simulink library "environments"  (R2014b)
settings: Solver=ode45  StartTime=0.0  StopTime=10.0  RelTol=1e-3
undefined symbols (not defined in the file): wheel, X, Y, Z
libraries: sm_lib x52, contactlibV2 x20, nesl_utility x4
settings Model: Creator=scastro  LastModifiedBy=scastro

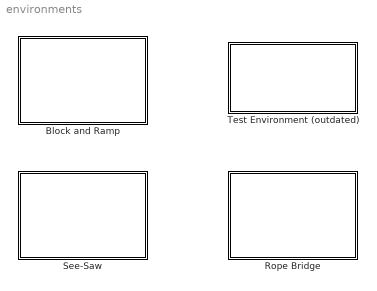
== system environments ==
  Block and Ramp : Subsystem  mask{k=3000, b=25, b2=10}
      mask prompts: k "Contact Stiffness"; b "Contact Damping"; b2 "Friction Damping"
  Rope Bridge : Subsystem  VariantControl=Variant2  mask{k=3000, b=25, b2=10, kbridge=10, dbridge=0.05}
      mask prompts: k "Contact Stiffness"; b "Contact Damping"; b2 "Friction Damping"; kbridge "Bridge Stiffness"; dbridge "Bridge Damping"
  See-Saw : Subsystem  mask{k=3000, b=25, b2=10}
      mask prompts: k "Contact Stiffness"; b "Contact Damping"; b2 "Friction Damping"
  Test Environment (outdated) : Subsystem

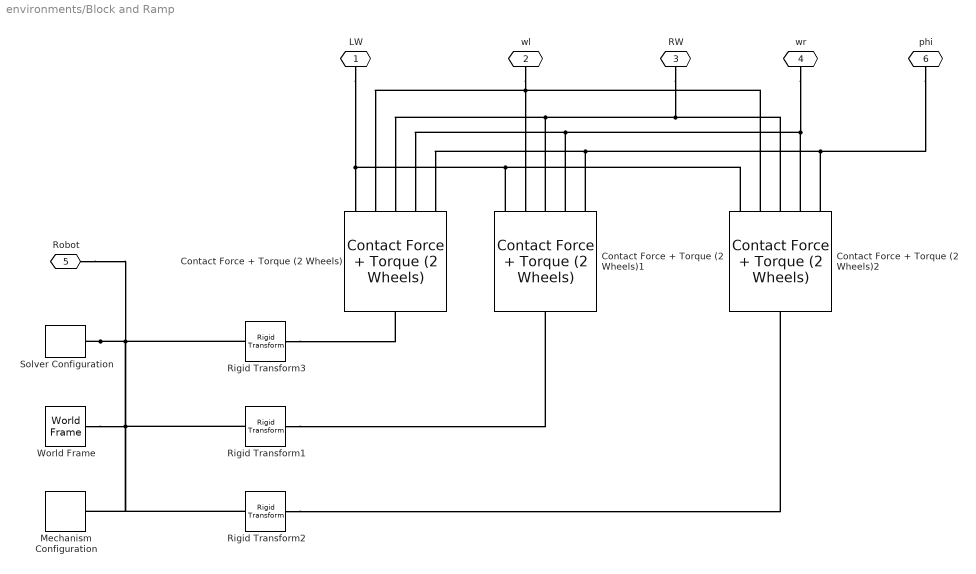
== system environments/Block and Ramp ==
  Contact Force + Torque (2 Wheels) : contactlibV2/Contact Force + Torque (2 Wheels)  rWheel=wheel.r  k=k  b=b  b2=b2  xBlock=3  yBlock=3  zBlock=0.01  mBlock=5  blockColor=[0.2 0.2 1]
  Contact Force + Torque (2 Wheels)1 : contactlibV2/Contact Force + Torque (2 Wheels)  rWheel=wheel.r  k=k  b=b  b2=b2  xBlock=1  yBlock=3  zBlock=0.025  mBlock=5  blockColor=[0.2 0.6 0.2]
  Contact Force + Torque (2 Wheels)2 : contactlibV2/Contact Force + Torque (2 Wheels)  rWheel=wheel.r  k=k  b=b  b2=b2  xBlock=1  yBlock=3  zBlock=0.025  mBlock=5  blockColor=[0.6 0.2 0.2]
  Mechanism Configuration : sm_lib/Utilities/Mechanism Configuration  UniformGravity=Constant  GravityVector=[0 0 -9.80665]  GravityUnits=m/s^2  LinearizationDelta=0.001  BlockFunction=simmechanics.library.utilities.mechanism_configuration
  Rigid Transform1 : sm_lib/Frames and Transforms/Rigid Transform  TranslationMethod=Cartesian  TranslationLengthUnit=m  TranslationStandardAxis=+Z  TranslationStandardOffset=0  TranslationCartesianOffset=[1 0 0.0825-0.12]  TranslationROffset=0  TranslationROffsetUnits=m  TranslationZOffset=0  TranslationZOffsetUnits=m  TranslationThetaOffset=0  TranslationThetaOffsetUnits=deg  RotationMethod=StandardAxis  RotationAngleUnits=deg  RotationStandardAxis=+Z  RotationAngle=0  RotationArbitraryAxis=[0 0 1]  FollAlignAxisA=+X  BaseAlignAxisA=+Y  FollAlignAxisB=+Y  BaseAlignAxisB=+Z  RotationMatrix=[1 0 0; 0 1 0; 0 0 1]  BlockFunction=simmechanics.library.frames_transforms.rigid_transform
  Rigid Transform2 : sm_lib/Frames and Transforms/Rigid Transform  TranslationMethod=Cartesian  TranslationLengthUnit=m  TranslationStandardAxis=+Z  TranslationStandardOffset=0  TranslationCartesianOffset=[-1 0 0.084]  TranslationROffset=0  TranslationROffsetUnits=m  TranslationZOffset=0  TranslationZOffsetUnits=m  TranslationThetaOffset=0  TranslationThetaOffsetUnits=deg  RotationMethod=StandardAxis  RotationAngleUnits=deg  RotationStandardAxis=+Y  RotationAngle=15  RotationArbitraryAxis=[0 0 1]  FollAlignAxisA=+X  BaseAlignAxisA=+Y  FollAlignAxisB=+Y  BaseAlignAxisB=+Z  RotationMatrix=[1 0 0; 0 1 0; 0 0 1]  BlockFunction=simmechanics.library.frames_transforms.rigid_transform
  Rigid Transform3 : sm_lib/Frames and Transforms/Rigid Transform  TranslationMethod=Cartesian  TranslationLengthUnit=m  TranslationStandardAxis=+Z  TranslationStandardOffset=0  TranslationCartesianOffset=[0 0 -(wheel.r+0.01)]  TranslationROffset=0  TranslationROffsetUnits=m  TranslationZOffset=0  TranslationZOffsetUnits=m  TranslationThetaOffset=0  TranslationThetaOffsetUnits=deg  RotationMethod=StandardAxis  RotationAngleUnits=deg  RotationStandardAxis=+Z  RotationAngle=0  RotationArbitraryAxis=[0 0 1]  FollAlignAxisA=+X  BaseAlignAxisA=+Y  FollAlignAxisB=+Y  BaseAlignAxisB=+Z  RotationMatrix=[1 0 0; 0 1 0; 0 0 1]  BlockFunction=simmechanics.library.frames_transforms.rigid_transform
  Solver Configuration : nesl_utility/Solver Configuration  PhysicalDomain=network_engine_domain  SubClassName=solver  LeftPortType=input  RightPortType=generic  Accelerate=off  Tones=[]  Harmonics=[]  SimulateNoise=off  Profile=off  UseLocalSampling=off  EnableSwitchedLinearOptims=on  FrequencyDomain=off  UseCCode=off  RelTol=0.001  AbsTol=1e-06  MinStep=1e-09  ToWorkspace=off  DoDC=off  ResidualTolerance=1e-09  UseLocalSolver=off  LocalSolverChoice=NE_BACKWARD_EULER_ADVANCER  LocalSolverSampleTime=0.001  DoFixedCost=off  MaxNonlinIter=3  MaxModeIter=2  LinearAlgebra=Sparse  DelaysMemoryBudget=1024  AutomaticFiltering=on  FilteringTimeConstant=0.001
  World Frame : sm_lib/Frames and Transforms/World Frame  BlockFunction=simmechanics.library.frames_transforms.world_frame
  LW : PMIOPort  Port=1  Side=Right
  wl : PMIOPort  Port=2  Side=Right
  RW : PMIOPort  Port=3  Side=Right
  wr : PMIOPort  Port=4  Side=Right
  Robot : PMIOPort  Port=5  Side=Left
  phi : PMIOPort  Port=6  Side=Right
  connections:
  Rigid Transform3/RConn1 -- Contact Force + Torque (2 Wheels)/LConn1
  Solver Configuration/RConn1 -- Rigid Transform1/LConn1 -- Mechanism Configuration/RConn1 -- Rigid Transform2/LConn1 -- World Frame/RConn1 -- Robot/RConn1 -- Rigid Transform3/LConn1
  Contact Force + Torque (2 Wheels)1/RConn1 -- Contact Force + Torque (2 Wheels)/RConn1 -- LW/RConn1 -- Contact Force + Torque (2 Wheels)2/RConn1
  Rigid Transform1/RConn1 -- Contact Force + Torque (2 Wheels)1/LConn1
  wl/RConn1 -- Contact Force + Torque (2 Wheels)2/RConn2 -- Contact Force + Torque (2 Wheels)1/RConn2 -- Contact Force + Torque (2 Wheels)/RConn2
  RW/RConn1 -- Contact Force + Torque (2 Wheels)2/RConn3 -- Contact Force + Torque (2 Wheels)1/RConn3 -- Contact Force + Torque (2 Wheels)/RConn3
  wr/RConn1 -- Contact Force + Torque (2 Wheels)2/RConn4 -- Contact Force + Torque (2 Wheels)1/RConn4 -- Contact Force + Torque (2 Wheels)/RConn4
  phi/RConn1 -- Contact Force + Torque (2 Wheels)2/RConn5 -- Contact Force + Torque (2 Wheels)1/RConn5 -- Contact Force + Torque (2 Wheels)/RConn5
  Rigid Transform2/RConn1 -- Contact Force + Torque (2 Wheels)2/LConn1

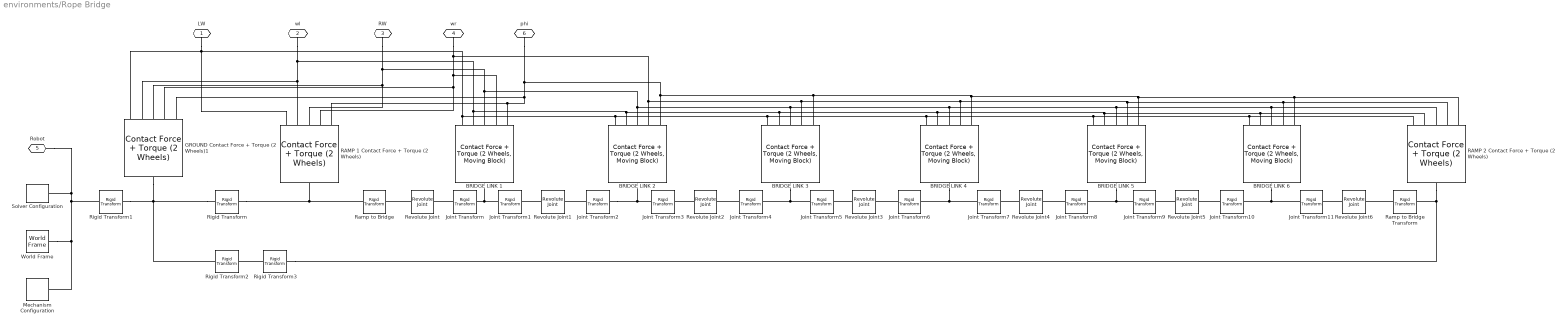
== system environments/Rope Bridge ==
  " BRIDGE LINK 1" : contactlibV2/Contact Force + Torque (2 Wheels, Moving Block)  rWheel=wheel.r  k=k  b=b  b2=b2  xBlock=2.5*(0.0254)  yBlock=12*(0.0254)  zBlock=0.75*(0.0254)  mBlock=0.2  blockColor=[1 0 0]
  " BRIDGE LINK 2" : contactlibV2/Contact Force + Torque (2 Wheels, Moving Block)  rWheel=wheel.r  k=k  b=b  b2=b2  xBlock=2.5*(0.0254)  yBlock=12*(0.0254)  zBlock=0.75*(0.0254)  mBlock=0.2  blockColor=[0 1 0]
  " BRIDGE LINK 3" : contactlibV2/Contact Force + Torque (2 Wheels, Moving Block)  rWheel=wheel.r  k=k  b=b  b2=b2  xBlock=2.5*(0.0254)  yBlock=12*(0.0254)  zBlock=0.75*(0.0254)  mBlock=0.2  blockColor=[1 0 0]
  " BRIDGE LINK 4" : contactlibV2/Contact Force + Torque (2 Wheels, Moving Block)  rWheel=wheel.r  k=k  b=b  b2=b2  xBlock=2.5*(0.0254)  yBlock=12*(0.0254)  zBlock=0.75*(0.0254)  mBlock=0.2  blockColor=[0 1 0]
  " BRIDGE LINK 5" : contactlibV2/Contact Force + Torque (2 Wheels, Moving Block)  rWheel=wheel.r  k=k  b=b  b2=b2  xBlock=2.5*(0.0254)  yBlock=12*(0.0254)  zBlock=0.75*(0.0254)  mBlock=0.2  blockColor=[1 0 0]
  " BRIDGE LINK 6" : contactlibV2/Contact Force + Torque (2 Wheels, Moving Block)  rWheel=wheel.r  k=k  b=b  b2=b2  xBlock=2.5*(0.0254)  yBlock=12*(0.0254)  zBlock=0.75*(0.0254)  mBlock=0.2  blockColor=[0 1 0]
  GROUND Contact Force + Torque (2 Wheels)1 : contactlibV2/Contact Force + Torque (2 Wheels)  rWheel=wheel.r  k=k  b=b  b2=b2  xBlock=24*(0.0254)  yBlock=12*(0.0254)  zBlock=0.5*(0.0254)  mBlock=5  blockColor=[0.2 0.2 0.6]
  Joint Transform : sm_lib/Frames and Transforms/Rigid Transform  TranslationMethod=StandardAxis  TranslationLengthUnit=in  TranslationStandardAxis=+X  TranslationStandardOffset=1.25  TranslationCartesianOffset=[1.25 0 -0.2]  TranslationROffset=0  TranslationROffsetUnits=m  TranslationZOffset=0  TranslationZOffsetUnits=m  TranslationThetaOffset=0  TranslationThetaOffsetUnits=deg  RotationMethod=StandardAxis  RotationAngleUnits=deg  RotationStandardAxis=-X  RotationAngle=90  RotationArbitraryAxis=[0 0 1]  FollAlignAxisA=+X  BaseAlignAxisA=+Y  FollAlignAxisB=+Y  BaseAlignAxisB=+Z  RotationMatrix=[1 0 0; 0 1 0; 0 0 1]  BlockFunction=simmechanics.library.frames_transforms.rigid_transform
  Joint Transform{1,3,5,7,9} (5 alike) : sm_lib/Frames and Transforms/Rigid Transform  TranslationMethod=StandardAxis  TranslationLengthUnit=in  TranslationStandardAxis=+X  TranslationStandardOffset=1.25  TranslationCartesianOffset=[(11*cos(asin(4.75/22))) 0 4.75/2]  TranslationROffset=0  TranslationROffsetUnits=m  TranslationZOffset=0  TranslationZOffsetUnits=m  TranslationThetaOffset=0  TranslationThetaOffsetUnits=deg  RotationMethod=StandardAxis  RotationAngleUnits=deg  RotationStandardAxis=+X  RotationAngle=90  RotationArbitraryAxis=[0 0 1]  FollAlignAxisA=+X  BaseAlignAxisA=+Y  FollAlignAxisB=+Y  BaseAlignAxisB=+Z  RotationMatrix=[1 0 0; 0 1 0; 0 0 1]  BlockFunction=simmechanics.library.frames_transforms.rigid_transform
  Joint Transform{2,4,6,8,10} (5 alike) : sm_lib/Frames and Transforms/Rigid Transform  TranslationMethod=StandardAxis  TranslationLengthUnit=in  TranslationStandardAxis=+X  TranslationStandardOffset=1.25  TranslationCartesianOffset=[(11*cos(asin(4.75/22))) 0 4.75/2]  TranslationROffset=0  TranslationROffsetUnits=m  TranslationZOffset=0  TranslationZOffsetUnits=m  TranslationThetaOffset=0  TranslationThetaOffsetUnits=deg  RotationMethod=StandardAxis  RotationAngleUnits=deg  RotationStandardAxis=-X  RotationAngle=90  RotationArbitraryAxis=[0 0 1]  FollAlignAxisA=+X  BaseAlignAxisA=+Y  FollAlignAxisB=+Y  BaseAlignAxisB=+Z  RotationMatrix=[1 0 0; 0 1 0; 0 0 1]  BlockFunction=simmechanics.library.frames_transforms.rigid_transform
  Joint Transform11 : sm_lib/Frames and Transforms/Rigid Transform  TranslationMethod=Cartesian  TranslationLengthUnit=in  TranslationStandardAxis=+X  TranslationStandardOffset=1.25  TranslationCartesianOffset=[1.25 0 0]  TranslationROffset=0  TranslationROffsetUnits=m  TranslationZOffset=0  TranslationZOffsetUnits=m  TranslationThetaOffset=0  TranslationThetaOffsetUnits=deg  RotationMethod=StandardAxis  RotationAngleUnits=deg  RotationStandardAxis=+X  RotationAngle=90  RotationArbitraryAxis=[0 0 1]  FollAlignAxisA=+X  BaseAlignAxisA=+Y  FollAlignAxisB=+Y  BaseAlignAxisB=+Z  RotationMatrix=[1 0 0; 0 1 0; 0 0 1]  BlockFunction=simmechanics.library.frames_transforms.rigid_transform
  Mechanism Configuration : sm_lib/Utilities/Mechanism Configuration  UniformGravity=Constant  GravityVector=[0 0 -9.80665]  GravityUnits=m/s^2  LinearizationDelta=0.001  BlockFunction=simmechanics.library.utilities.mechanism_configuration
  RAMP 1 Contact Force + Torque (2 Wheels) : contactlibV2/Contact Force + Torque (2 Wheels)  rWheel=wheel.r  k=k  b=b  b2=b2  xBlock=22*(0.0254)  yBlock=12*(0.0254)  zBlock=0.5*(0.0254)  mBlock=5  blockColor=[0.2 0.2 1]
  RAMP 2 Contact Force + Torque (2 Wheels) : contactlibV2/Contact Force + Torque (2 Wheels)  rWheel=wheel.r  k=k  b=b  b2=b2  xBlock=24*(0.0254)  yBlock=12*(0.0254)  zBlock=0.5*(0.0254)  mBlock=5  blockColor=[0.2 0.2 0.6]
  Ramp to Bridge : sm_lib/Frames and Transforms/Rigid Transform  TranslationMethod=Cartesian  TranslationLengthUnit=in  TranslationStandardAxis=+X  TranslationStandardOffset=11  TranslationCartesianOffset=[11 0 -0.1]  TranslationROffset=0  TranslationROffsetUnits=m  TranslationZOffset=0  TranslationZOffsetUnits=m  TranslationThetaOffset=0  TranslationThetaOffsetUnits=deg  RotationMethod=StandardAxis  RotationAngleUnits=deg  RotationStandardAxis=+X  RotationAngle=90  RotationArbitraryAxis=[0 0 1]  FollAlignAxisA=+X  BaseAlignAxisA=+Y  FollAlignAxisB=+Y  BaseAlignAxisB=+Z  RotationMatrix=[1 0 0; 0 1 0; 0 0 1]  BlockFunction=simmechanics.library.frames_transforms.rigid_transform
  Ramp to Bridge Transform : sm_lib/Frames and Transforms/Rigid Transform  TranslationMethod=Cartesian  TranslationLengthUnit=in  TranslationStandardAxis=-X  TranslationStandardOffset=12  TranslationCartesianOffset=[-12 0 -0.1]  TranslationROffset=0  TranslationROffsetUnits=m  TranslationZOffset=0  TranslationZOffsetUnits=m  TranslationThetaOffset=0  TranslationThetaOffsetUnits=deg  RotationMethod=StandardAxis  RotationAngleUnits=deg  RotationStandardAxis=+X  RotationAngle=90  RotationArbitraryAxis=[0 0 1]  FollAlignAxisA=+X  BaseAlignAxisA=+Y  FollAlignAxisB=+Y  BaseAlignAxisB=+Z  RotationMatrix=[1 0 0; 0 1 0; 0 0 1]  BlockFunction=simmechanics.library.frames_transforms.rigid_transform
  Revolute Joint{,1..6} (7 alike) : sm_lib/Joints/Revolute Joint  SenseConstraintForce=off  SenseConstraintForceX=off  SenseConstraintForceY=off  SenseConstraintForceZ=off  SenseConstraintTorque=off  SenseConstraintTorqueX=off  SenseConstraintTorqueY=off  SenseConstraintTorqueZ=off  SenseTotalForce=off  SenseTotalForceX=off  SenseTotalForceY=off  SenseTotalForceZ=off  SenseTotalTorque=off  SenseTotalTorqueX=off  SenseTotalTorqueY=off  SenseTotalTorqueZ=off  CompositeWrenchDir=FollowerOnBase  CompositeWrenchFrame=BaseFrame  EquilibriumPosition=0  EquilibriumPositionUnits=deg  SpringStiffness=kbridge  SpringStiffnessUnits=N*m/rad  DampingCoefficient=dbridge  DampingCoefficientUnits=N*m/(rad/s)  TorqueActuationMode=NoTorque  MotionActuationMode=ComputedMotion  SensePosition=off  SenseVelocity=off  SenseAcceleration=off  SenseTorqueForce=off  PositionTargetValue=0  PositionTargetValueUnits=deg  PositionTargetSpecify=off  PositionTargetPriority=High  VelocityTargetValue=0  VelocityTargetValueUnits=deg/s  VelocityTargetSpecify=off  VelocityTargetPriority=High  BlockFunction=simmechanics.library.joints.revolute_joint
  Rigid Transform : sm_lib/Frames and Transforms/Rigid Transform  TranslationMethod=Cartesian  TranslationLengthUnit=in  TranslationStandardAxis=+Z  TranslationStandardOffset=0  TranslationCartesianOffset=[(12+11*cos(asin(4.75/22))) 0 4.75/2]  TranslationROffset=0  TranslationROffsetUnits=m  TranslationZOffset=0  TranslationZOffsetUnits=m  TranslationThetaOffset=0  TranslationThetaOffsetUnits=deg  RotationMethod=StandardAxis  RotationAngleUnits=rad  RotationStandardAxis=+Y  RotationAngle=-asin(4.75/22)  RotationArbitraryAxis=[0 0 1]  FollAlignAxisA=+X  BaseAlignAxisA=+Y  FollAlignAxisB=+Y  BaseAlignAxisB=+Z  RotationMatrix=[1 0 0; 0 1 0; 0 0 1]  BlockFunction=simmechanics.library.frames_transforms.rigid_transform
  Rigid Transform1 : sm_lib/Frames and Transforms/Rigid Transform  TranslationMethod=Cartesian  TranslationLengthUnit=m  TranslationStandardAxis=+Z  TranslationStandardOffset=0  TranslationCartesianOffset=[0 0.1 -0.05]  TranslationROffset=0  TranslationROffsetUnits=m  TranslationZOffset=0  TranslationZOffsetUnits=m  TranslationThetaOffset=0  TranslationThetaOffsetUnits=deg  RotationMethod=None  RotationAngleUnits=rad  RotationStandardAxis=+Y  RotationAngle=-asin(4.75/22)  RotationArbitraryAxis=[0 0 1]  FollAlignAxisA=+X  BaseAlignAxisA=+Y  FollAlignAxisB=+Y  BaseAlignAxisB=+Z  RotationMatrix=[1 0 0; 0 1 0; 0 0 1]  BlockFunction=simmechanics.library.frames_transforms.rigid_transform
  Rigid Transform2 : sm_lib/Frames and Transforms/Rigid Transform  TranslationMethod=Cartesian  TranslationLengthUnit=in  TranslationStandardAxis=+Z  TranslationStandardOffset=0  TranslationCartesianOffset=[(12+ 22*cos(asin(4.75/22)) + 14.5 + 12*cos(asin(5.875/24)) ) 0 (4.75+ (5.875/2))]  TranslationROffset=0  TranslationROffsetUnits=m  TranslationZOffset=0  TranslationZOffsetUnits=m  TranslationThetaOffset=0  TranslationThetaOffsetUnits=deg  RotationMethod=None  RotationAngleUnits=rad  RotationStandardAxis=+Y  RotationAngle=-asin(4.75/22)  RotationArbitraryAxis=[0 0 1]  FollAlignAxisA=+X  BaseAlignAxisA=+Y  FollAlignAxisB=+Y  BaseAlignAxisB=+Z  RotationMatrix=[1 0 0; 0 1 0; 0 0 1]  BlockFunction=simmechanics.library.frames_transforms.rigid_transform
  Rigid Transform3 : sm_lib/Frames and Transforms/Rigid Transform  TranslationMethod=None  TranslationLengthUnit=in  TranslationStandardAxis=+Z  TranslationStandardOffset=0  TranslationCartesianOffset=[(12+ 11*cos(asin(4.75/22)) + 14.5 + 12*cos(asin(5.875/24)) ) 0 (4.75+5.875)/2]  TranslationROffset=0  TranslationROffsetUnits=m  TranslationZOffset=0  TranslationZOffsetUnits=m  TranslationThetaOffset=0  TranslationThetaOffsetUnits=deg  RotationMethod=StandardAxis  RotationAngleUnits=rad  RotationStandardAxis=+Y  RotationAngle=-asin(5.875/24)  RotationArbitraryAxis=[0 0 1]  FollAlignAxisA=+X  BaseAlignAxisA=+Y  FollAlignAxisB=+Y  BaseAlignAxisB=+Z  RotationMatrix=[1 0 0; 0 1 0; 0 0 1]  BlockFunction=simmechanics.library.frames_transforms.rigid_transform
  Solver Configuration : nesl_utility/Solver Configuration  PhysicalDomain=network_engine_domain  SubClassName=solver  LeftPortType=input  RightPortType=generic  Accelerate=off  Tones=[]  Harmonics=[]  SimulateNoise=off  Profile=off  UseLocalSampling=off  EnableSwitchedLinearOptims=on  FrequencyDomain=off  UseCCode=off  RelTol=0.001  AbsTol=1e-06  MinStep=1e-09  ToWorkspace=off  DoDC=off  ResidualTolerance=1e-09  UseLocalSolver=off  LocalSolverChoice=NE_BACKWARD_EULER_ADVANCER  LocalSolverSampleTime=0.001  DoFixedCost=off  MaxNonlinIter=3  MaxModeIter=2  LinearAlgebra=Sparse  DelaysMemoryBudget=1024  AutomaticFiltering=on  FilteringTimeConstant=0.001
  World Frame : sm_lib/Frames and Transforms/World Frame  BlockFunction=simmechanics.library.frames_transforms.world_frame
  LW : PMIOPort  Port=1  Side=Right
  wl : PMIOPort  Port=2  Side=Right
  RW : PMIOPort  Port=3  Side=Right
  wr : PMIOPort  Port=4  Side=Right
  Robot : PMIOPort  Port=5  Side=Left
  phi : PMIOPort  Port=6  Side=Right
  connections:
  " BRIDGE LINK 5"/RConn5 -- " BRIDGE LINK 4"/RConn5 -- " BRIDGE LINK 3"/RConn5 -- " BRIDGE LINK 2"/RConn5 -- phi/RConn1 -- GROUND Contact Force + Torque (2 Wheels)1/RConn5 -- " BRIDGE LINK 1"/RConn5 -- RAMP 1 Contact Force + Torque (2 Wheels)/RConn5 -- " BRIDGE LINK 6"/RConn5 -- RAMP 2 Contact Force + Torque (2 Wheels)/RConn5
  " BRIDGE LINK 5"/RConn4 -- " BRIDGE LINK 4"/RConn4 -- " BRIDGE LINK 3"/RConn4 -- " BRIDGE LINK 2"/RConn4 -- wr/RConn1 -- " BRIDGE LINK 1"/RConn4 -- GROUND Contact Force + Torque (2 Wheels)1/RConn4 -- RAMP 1 Contact Force + Torque (2 Wheels)/RConn4 -- RAMP 2 Contact Force + Torque (2 Wheels)/RConn4 -- " BRIDGE LINK 6"/RConn4
  " BRIDGE LINK 5"/RConn3 -- " BRIDGE LINK 4"/RConn3 -- " BRIDGE LINK 3"/RConn3 -- " BRIDGE LINK 2"/RConn3 -- " BRIDGE LINK 1"/RConn3 -- RW/RConn1 -- GROUND Contact Force + Torque (2 Wheels)1/RConn3 -- RAMP 1 Contact Force + Torque (2 Wheels)/RConn3 -- RAMP 2 Contact Force + Torque (2 Wheels)/RConn3 -- " BRIDGE LINK 6"/RConn3
  " BRIDGE LINK 5"/RConn2 -- " BRIDGE LINK 4"/RConn2 -- " BRIDGE LINK 3"/RConn2 -- " BRIDGE LINK 2"/RConn2 -- " BRIDGE LINK 1"/RConn2 -- wl/RConn1 -- GROUND Contact Force + Torque (2 Wheels)1/RConn2 -- RAMP 1 Contact Force + Torque (2 Wheels)/RConn2 -- RAMP 2 Contact Force + Torque (2 Wheels)/RConn2 -- " BRIDGE LINK 6"/RConn2
  " BRIDGE LINK 5"/RConn1 -- " BRIDGE LINK 4"/RConn1 -- " BRIDGE LINK 3"/RConn1 -- " BRIDGE LINK 2"/RConn1 -- " BRIDGE LINK 1"/RConn1 -- GROUND Contact Force + Torque (2 Wheels)1/RConn1 -- LW/RConn1 -- RAMP 1 Contact Force + Torque (2 Wheels)/RConn1 -- RAMP 2 Contact Force + Torque (2 Wheels)/RConn1 -- " BRIDGE LINK 6"/RConn1
  Robot/RConn1 -- Solver Configuration/RConn1 -- World Frame/RConn1 -- Mechanism Configuration/RConn1 -- Rigid Transform1/LConn1
  Ramp to Bridge/LConn1 -- Rigid Transform/RConn1 -- RAMP 1 Contact Force + Torque (2 Wheels)/LConn1
  Rigid Transform/LConn1 -- GROUND Contact Force + Torque (2 Wheels)1/LConn1 -- Rigid Transform1/RConn1 -- Rigid Transform2/LConn1
  Joint Transform/RConn1 -- " BRIDGE LINK 1"/LConn1 -- Joint Transform1/LConn1
  Revolute Joint/LConn1 -- Ramp to Bridge/RConn1
  Joint Transform/LConn1 -- Revolute Joint/RConn1
  Revolute Joint1/LConn1 -- Joint Transform1/RConn1
  Joint Transform3/LConn1 -- Joint Transform2/RConn1 -- " BRIDGE LINK 2"/LConn1
  Joint Transform2/LConn1 -- Revolute Joint1/RConn1
  Joint Transform4/LConn1 -- Revolute Joint2/RConn1
  Revolute Joint2/LConn1 -- Joint Transform3/RConn1
  " BRIDGE LINK 3"/LConn1 -- Joint Transform4/RConn1 -- Joint Transform5/LConn1
  " BRIDGE LINK 4"/LConn1 -- Joint Transform6/RConn1 -- Joint Transform7/LConn1
  Revolute Joint3/LConn1 -- Joint Transform5/RConn1
  Joint Transform6/LConn1 -- Revolute Joint3/RConn1
  Joint Transform8/LConn1 -- Revolute Joint4/RConn1
  Revolute Joint4/LConn1 -- Joint Transform7/RConn1
  " BRIDGE LINK 5"/LConn1 -- Joint Transform8/RConn1 -- Joint Transform9/LConn1
  Revolute Joint5/LConn1 -- Joint Transform9/RConn1
  " BRIDGE LINK 6"/LConn1 -- Joint Transform10/RConn1 -- Joint Transform11/LConn1
  Joint Transform10/LConn1 -- Revolute Joint5/RConn1
  Revolute Joint6/LConn1 -- Joint Transform11/RConn1
  Ramp to Bridge Transform/LConn1 -- RAMP 2 Contact Force + Torque (2 Wheels)/LConn1 -- Rigid Transform3/RConn1
  Ramp to Bridge Transform/RConn1 -- Revolute Joint6/RConn1
  Rigid Transform3/LConn1 -- Rigid Transform2/RConn1

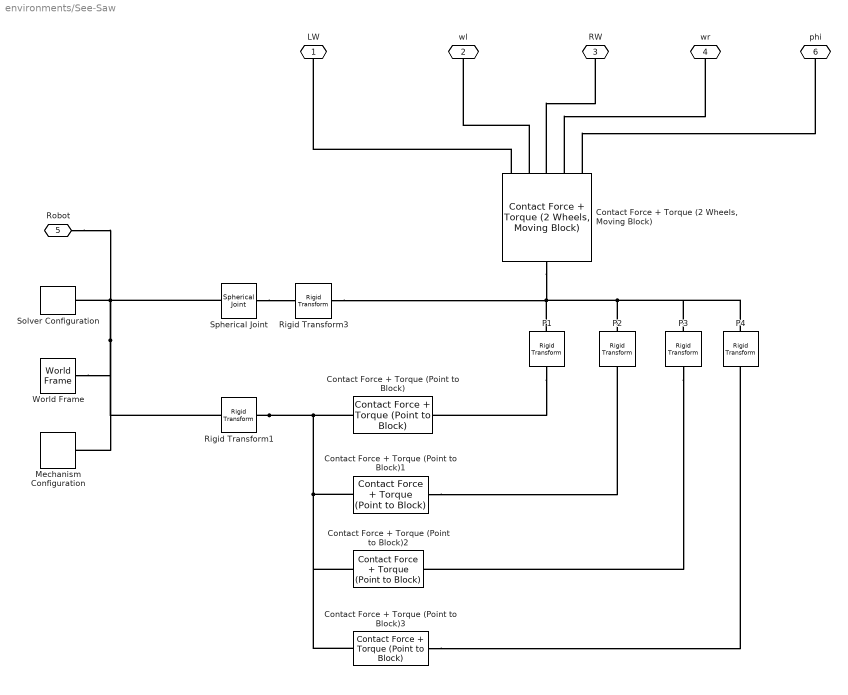
== system environments/See-Saw ==
  "Contact Force + Torque (2 Wheels, Moving Block)" : contactlibV2/Contact Force + Torque (2 Wheels, Moving Block)  rWheel=wheel.r  k=k  b=b  b2=b2  xBlock=2  yBlock=2  zBlock=0.01  mBlock=5  blockColor=[0.2 0.2 1]
  Contact Force + Torque (Point to Block){,1..3} (4 alike) : contactlibV2/Contact Force + Torque (Point to Block)  k=k  b=b  xBlock=5  yBlock=5  zBlock=0.01  mBlock=5  blockColor=[0.2 1 0.2]
  Mechanism Configuration : sm_lib/Utilities/Mechanism Configuration  UniformGravity=Constant  GravityVector=[0 0 -9.80665]  GravityUnits=m/s^2  LinearizationDelta=0.001  BlockFunction=simmechanics.library.utilities.mechanism_configuration
  P1 : sm_lib/Frames and Transforms/Rigid Transform  TranslationMethod=Cartesian  TranslationLengthUnit=m  TranslationStandardAxis=+Z  TranslationStandardOffset=0  TranslationCartesianOffset=[-1 -1 -0.005]  TranslationROffset=0  TranslationROffsetUnits=m  TranslationZOffset=0  TranslationZOffsetUnits=m  TranslationThetaOffset=0  TranslationThetaOffsetUnits=deg  RotationMethod=None  RotationAngleUnits=deg  RotationStandardAxis=-X  RotationAngle=90  RotationArbitraryAxis=[0 0 1]  FollAlignAxisA=+X  BaseAlignAxisA=+Y  FollAlignAxisB=+Y  BaseAlignAxisB=+Z  BlockFunction=simmechanics.library.frames_transforms.rigid_transform
  P2 : sm_lib/Frames and Transforms/Rigid Transform  TranslationMethod=Cartesian  TranslationLengthUnit=m  TranslationStandardAxis=+Z  TranslationStandardOffset=0  TranslationCartesianOffset=[-1 1 -0.005]  TranslationROffset=0  TranslationROffsetUnits=m  TranslationZOffset=0  TranslationZOffsetUnits=m  TranslationThetaOffset=0  TranslationThetaOffsetUnits=deg  RotationMethod=None  RotationAngleUnits=deg  RotationStandardAxis=-X  RotationAngle=90  RotationArbitraryAxis=[0 0 1]  FollAlignAxisA=+X  BaseAlignAxisA=+Y  FollAlignAxisB=+Y  BaseAlignAxisB=+Z  BlockFunction=simmechanics.library.frames_transforms.rigid_transform
  P3 : sm_lib/Frames and Transforms/Rigid Transform  TranslationMethod=Cartesian  TranslationLengthUnit=m  TranslationStandardAxis=+Z  TranslationStandardOffset=0  TranslationCartesianOffset=[1 -1 -0.005]  TranslationROffset=0  TranslationROffsetUnits=m  TranslationZOffset=0  TranslationZOffsetUnits=m  TranslationThetaOffset=0  TranslationThetaOffsetUnits=deg  RotationMethod=None  RotationAngleUnits=deg  RotationStandardAxis=-X  RotationAngle=90  RotationArbitraryAxis=[0 0 1]  FollAlignAxisA=+X  BaseAlignAxisA=+Y  FollAlignAxisB=+Y  BaseAlignAxisB=+Z  BlockFunction=simmechanics.library.frames_transforms.rigid_transform
  P4 : sm_lib/Frames and Transforms/Rigid Transform  TranslationMethod=Cartesian  TranslationLengthUnit=m  TranslationStandardAxis=+Z  TranslationStandardOffset=0  TranslationCartesianOffset=[1 1 -0.005]  TranslationROffset=0  TranslationROffsetUnits=m  TranslationZOffset=0  TranslationZOffsetUnits=m  TranslationThetaOffset=0  TranslationThetaOffsetUnits=deg  RotationMethod=None  RotationAngleUnits=deg  RotationStandardAxis=-X  RotationAngle=90  RotationArbitraryAxis=[0 0 1]  FollAlignAxisA=+X  BaseAlignAxisA=+Y  FollAlignAxisB=+Y  BaseAlignAxisB=+Z  BlockFunction=simmechanics.library.frames_transforms.rigid_transform
  Rigid Transform1 : sm_lib/Frames and Transforms/Rigid Transform  TranslationMethod=Cartesian  TranslationLengthUnit=m  TranslationStandardAxis=+Z  TranslationStandardOffset=0  TranslationCartesianOffset=[0 0 -0.2]  TranslationROffset=0  TranslationROffsetUnits=m  TranslationZOffset=0  TranslationZOffsetUnits=m  TranslationThetaOffset=0  TranslationThetaOffsetUnits=deg  RotationMethod=None  RotationAngleUnits=deg  RotationStandardAxis=-X  RotationAngle=90  RotationArbitraryAxis=[0 0 1]  FollAlignAxisA=+X  BaseAlignAxisA=+Y  FollAlignAxisB=+Y  BaseAlignAxisB=+Z  RotationMatrix=[1 0 0; 0 1 0; 0 0 1]  BlockFunction=simmechanics.library.frames_transforms.rigid_transform
  Rigid Transform3 : sm_lib/Frames and Transforms/Rigid Transform  TranslationMethod=Cartesian  TranslationLengthUnit=m  TranslationStandardAxis=+Z  TranslationStandardOffset=0  TranslationCartesianOffset=[0 0 -(wheel.r+0.01)]  TranslationROffset=0  TranslationROffsetUnits=m  TranslationZOffset=0  TranslationZOffsetUnits=m  TranslationThetaOffset=0  TranslationThetaOffsetUnits=deg  RotationMethod=None  RotationAngleUnits=deg  RotationStandardAxis=-X  RotationAngle=90  RotationArbitraryAxis=[0 0 1]  FollAlignAxisA=+X  BaseAlignAxisA=+Y  FollAlignAxisB=+Y  BaseAlignAxisB=+Z  BlockFunction=simmechanics.library.frames_transforms.rigid_transform
  Solver Configuration : nesl_utility/Solver Configuration  PhysicalDomain=network_engine_domain  SubClassName=solver  LeftPortType=input  RightPortType=generic  Accelerate=off  Tones=[]  Harmonics=[]  SimulateNoise=off  Profile=off  UseLocalSampling=off  EnableSwitchedLinearOptims=on  FrequencyDomain=off  UseCCode=off  RelTol=0.001  AbsTol=1e-06  MinStep=1e-09  ToWorkspace=off  DoDC=off  ResidualTolerance=1e-09  UseLocalSolver=off  LocalSolverChoice=NE_BACKWARD_EULER_ADVANCER  LocalSolverSampleTime=0.001  DoFixedCost=off  MaxNonlinIter=3  MaxModeIter=2  LinearAlgebra=Sparse  DelaysMemoryBudget=1024  AutomaticFiltering=on  FilteringTimeConstant=0.001
  Spherical Joint : sm_lib/Joints/Spherical Joint  SenseConstraintForce=off  SenseConstraintForceX=off  SenseConstraintForceY=off  SenseConstraintForceZ=off  SenseConstraintTorque=off  SenseConstraintTorqueX=off  SenseConstraintTorqueY=off  SenseConstraintTorqueZ=off  SenseTotalForce=off  SenseTotalForceX=off  SenseTotalForceY=off  SenseTotalForceZ=off  SenseTotalTorque=off  SenseTotalTorqueX=off  SenseTotalTorqueY=off  SenseTotalTorqueZ=off  CompositeWrenchDir=FollowerOnBase  CompositeWrenchFrame=BaseFrame  DefPosRotationMethod=None  DefPosRotationAngleUnits=deg  DefPosRotationStandardAxis=+Z  DefPosRotationAngle=0  DefPosRotationArbitraryAxis=[0 0 1]  DefPosFollAlignAxisA=+X  DefPosBaseAlignAxisA=+Y  DefPosFollAlignAxisB=+Y  DefPosBaseAlignAxisB=+Z  DefPosRotationMatrix=[1 0 0; 0 1 0; 0 0 1]  EqPosRotationMethod=None  EqPosRotationAngleUnits=deg  EqPosRotationStandardAxis=+Z  EqPosRotationAngle=0  EqPosRotationArbitraryAxis=[0 0 1]  EqPosFollAlignAxisA=+X  EqPosBaseAlignAxisA=+Y  EqPosFollAlignAxisB=+Y  EqPosBaseAlignAxisB=+Z  EqPosRotationMatrix=[1 0 0; 0 1 0; 0 0 1]  SpringStiffness=12  SpringStiffnessUnits=N*m/rad  DampingCoefficient=1.5  DampingCoefficientUnits=N*m/(rad/s)  ActuateTorqueX=off  ActuateTorqueY=off  ActuateTorqueZ=off  ActuateTorque=off  TorqueActuationMode=NoTorque  MotionActuationMode=ComputedMotion  ActuationFrame=BaseFrame  SensePosition=off  SenseVelocityX=off  SenseVelocityY=off  SenseVelocityZ=off  SenseVelocity=off  SenseAccelerationX=off  SenseAccelerationY=off  SenseAccelerationZ=off  SenseAcceleration=off  SenseTorqueX=off  SenseTorqueY=off  SenseTorqueZ=off  SenseTorqueForce=off  SensingFrame=BaseFrame  PositionTargetRotationMethod=None  PositionTargetRotationAngleUnits=deg  PositionTargetRotationStandardAxis=+Z  PositionTargetRotationAngle=0  PositionTargetRotationArbitraryAxis=[0 0 1]  PositionTargetFollAlignAxisA=+X  PositionTargetBaseAlignAxisA=+Y  PositionTargetFollAlignAxisB=+Y  PositionTargetBaseAlignAxisB=+Z  PositionTargetRotationMatrix=[1 0 0; 0 1 0; 0 0 1]  PositionTargetSpecify=off  PositionTargetPriority=High  VelocityTargetValue=[0 0 0]  VelocityTargetValueUnits=deg/s  VelocityTargetSpecify=off  VelocityTargetPriority=High  VelocityTargetInFollowerFrame=on  BlockFunction=simmechanics.library.joints.spherical_joint
  World Frame : sm_lib/Frames and Transforms/World Frame  BlockFunction=simmechanics.library.frames_transforms.world_frame
  LW : PMIOPort  Port=1  Side=Right
  wl : PMIOPort  Port=2  Side=Right
  RW : PMIOPort  Port=3  Side=Right
  wr : PMIOPort  Port=4  Side=Right
  Robot : PMIOPort  Port=5  Side=Left
  phi : PMIOPort  Port=6  Side=Right
  connections:
  "Contact Force + Torque (2 Wheels, Moving Block)"/RConn5 -- phi/RConn1
  "Contact Force + Torque (2 Wheels, Moving Block)"/RConn4 -- wr/RConn1
  "Contact Force + Torque (2 Wheels, Moving Block)"/RConn3 -- RW/RConn1
  "Contact Force + Torque (2 Wheels, Moving Block)"/RConn2 -- wl/RConn1
  "Contact Force + Torque (2 Wheels, Moving Block)"/RConn1 -- LW/RConn1
  Rigid Transform3/RConn1 -- P4/LConn1 -- P3/LConn1 -- P2/LConn1 -- P1/LConn1 -- "Contact Force + Torque (2 Wheels, Moving Block)"/LConn1
  Robot/RConn1 -- Spherical Joint/LConn1 -- World Frame/RConn1 -- Rigid Transform1/LConn1 -- Mechanism Configuration/RConn1 -- Solver Configuration/RConn1
  Spherical Joint/RConn1 -- Rigid Transform3/LConn1
  Rigid Transform1/RConn1 -- Contact Force + Torque (Point to Block)2/LConn1 -- Contact Force + Torque (Point to Block)3/LConn1 -- Contact Force + Torque (Point to Block)1/LConn1 -- Contact Force + Torque (Point to Block)/LConn1
  P1/RConn1 -- Contact Force + Torque (Point to Block)/RConn1
  Contact Force + Torque (Point to Block)1/RConn1 -- P2/RConn1
  P3/RConn1 -- Contact Force + Torque (Point to Block)2/RConn1
  Contact Force + Torque (Point to Block)3/RConn1 -- P4/RConn1

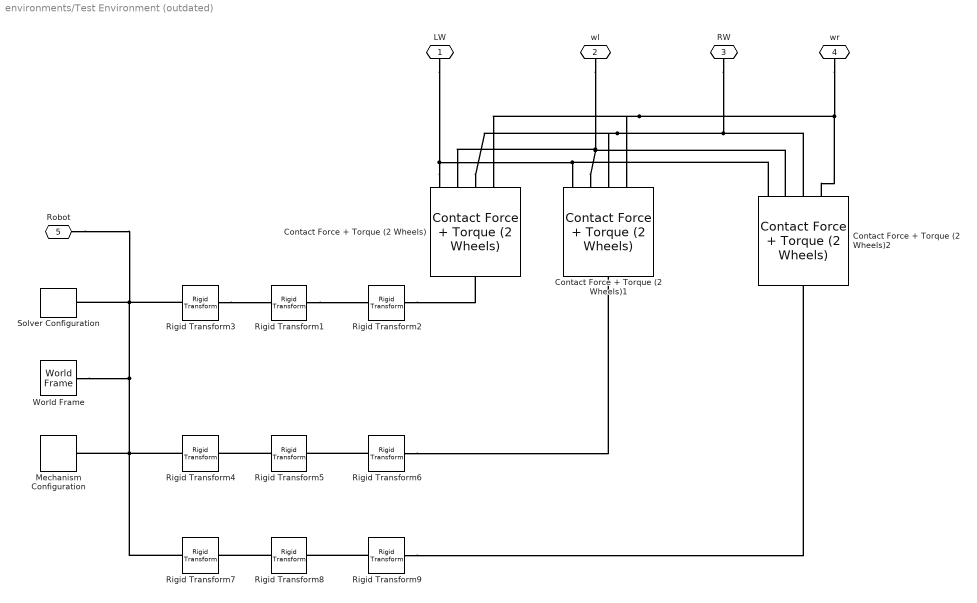
== system environments/Test Environment (outdated) ==
  Contact Force + Torque (2 Wheels) : contactlibV2/Contact Force + Torque (2 Wheels)  rWheel=wheel.r  k=1500  b=25  b2=10  xBlock=3  yBlock=3  zBlock=0.01  mBlock=5  blockColor=[0.2 0.2 1]
  Contact Force + Torque (2 Wheels)1 : contactlibV2/Contact Force + Torque (2 Wheels)  rWheel=wheel.r  k=1500  b=25  b2=10  xBlock=3  yBlock=3  zBlock=0.01  mBlock=5  blockColor=[1 0.2 0.2]
  Contact Force + Torque (2 Wheels)2 : contactlibV2/Contact Force + Torque (2 Wheels)  rWheel=wheel.r  k=1500  b=25  b2=10  xBlock=3  yBlock=3  zBlock=0.01  mBlock=5  blockColor=[0.2 1 0.2]
  Mechanism Configuration : sm_lib/Utilities/Mechanism Configuration  UniformGravity=Constant  GravityVector=[0 0 -9.80665]  GravityUnits=m/s^2  LinearizationDelta=0.001  BlockFunction=simmechanics.library.utilities.mechanism_configuration
  Rigid Transform1 : sm_lib/Frames and Transforms/Rigid Transform  TranslationMethod=None  TranslationLengthUnit=m  TranslationStandardAxis=+Z  TranslationStandardOffset=0  TranslationCartesianOffset=[0 0 -1.25]  TranslationROffset=0  TranslationROffsetUnits=m  TranslationZOffset=0  TranslationZOffsetUnits=m  TranslationThetaOffset=0  TranslationThetaOffsetUnits=deg  RotationMethod=StandardAxis  RotationAngleUnits=deg  RotationStandardAxis=+Y  RotationAngle=5  RotationArbitraryAxis=[0 0 1]  FollAlignAxisA=+X  BaseAlignAxisA=+Y  FollAlignAxisB=+Y  BaseAlignAxisB=+Z  BlockFunction=simmechanics.library.frames_transforms.rigid_transform
  Rigid Transform2 : sm_lib/Frames and Transforms/Rigid Transform  TranslationMethod=None  TranslationLengthUnit=m  TranslationStandardAxis=+Z  TranslationStandardOffset=0  TranslationCartesianOffset=[0 0 -1.25]  TranslationROffset=0  TranslationROffsetUnits=m  TranslationZOffset=0  TranslationZOffsetUnits=m  TranslationThetaOffset=0  TranslationThetaOffsetUnits=deg  RotationMethod=StandardAxis  RotationAngleUnits=deg  RotationStandardAxis=+X  RotationAngle=0  RotationArbitraryAxis=[0 0 1]  FollAlignAxisA=+X  BaseAlignAxisA=+Y  FollAlignAxisB=+Y  BaseAlignAxisB=+Z  BlockFunction=simmechanics.library.frames_transforms.rigid_transform
  Rigid Transform3 : sm_lib/Frames and Transforms/Rigid Transform  TranslationMethod=Cartesian  TranslationLengthUnit=m  TranslationStandardAxis=+Z  TranslationStandardOffset=0  TranslationCartesianOffset=[0 0 -(wheel.r+0.01)]  TranslationROffset=0  TranslationROffsetUnits=m  TranslationZOffset=0  TranslationZOffsetUnits=m  TranslationThetaOffset=0  TranslationThetaOffsetUnits=deg  RotationMethod=StandardAxis  RotationAngleUnits=deg  RotationStandardAxis=+Z  RotationAngle=0  RotationArbitraryAxis=[0 0 1]  FollAlignAxisA=+X  BaseAlignAxisA=+Y  FollAlignAxisB=+Y  BaseAlignAxisB=+Z  RotationMatrix=[1 0 0; 0 1 0; 0 0 1]  BlockFunction=simmechanics.library.frames_transforms.rigid_transform
  Rigid Transform4 : sm_lib/Frames and Transforms/Rigid Transform  TranslationMethod=Cartesian  TranslationLengthUnit=m  TranslationStandardAxis=+Z  TranslationStandardOffset=0  TranslationCartesianOffset=[3 -0 -0.35]  TranslationROffset=0  TranslationROffsetUnits=m  TranslationZOffset=0  TranslationZOffsetUnits=m  TranslationThetaOffset=0  TranslationThetaOffsetUnits=deg  RotationMethod=StandardAxis  RotationAngleUnits=deg  RotationStandardAxis=+Z  RotationAngle=115  RotationArbitraryAxis=[0 0 1]  FollAlignAxisA=+X  BaseAlignAxisA=+Y  FollAlignAxisB=+Y  BaseAlignAxisB=+Z  RotationMatrix=[1 0 0; 0 1 0; 0 0 1]  BlockFunction=simmechanics.library.frames_transforms.rigid_transform
  Rigid Transform5 : sm_lib/Frames and Transforms/Rigid Transform  TranslationMethod=None  TranslationLengthUnit=m  TranslationStandardAxis=+Z  TranslationStandardOffset=0  TranslationCartesianOffset=[0 0 -1.25]  TranslationROffset=0  TranslationROffsetUnits=m  TranslationZOffset=0  TranslationZOffsetUnits=m  TranslationThetaOffset=0  TranslationThetaOffsetUnits=deg  RotationMethod=StandardAxis  RotationAngleUnits=deg  RotationStandardAxis=+Y  RotationAngle=-1  RotationArbitraryAxis=[0 0 1]  FollAlignAxisA=+X  BaseAlignAxisA=+Y  FollAlignAxisB=+Y  BaseAlignAxisB=+Z  BlockFunction=simmechanics.library.frames_transforms.rigid_transform
  Rigid Transform6 : sm_lib/Frames and Transforms/Rigid Transform  TranslationMethod=None  TranslationLengthUnit=m  TranslationStandardAxis=+Z  TranslationStandardOffset=0  TranslationCartesianOffset=[0 0 -1.25]  TranslationROffset=0  TranslationROffsetUnits=m  TranslationZOffset=0  TranslationZOffsetUnits=m  TranslationThetaOffset=0  TranslationThetaOffsetUnits=deg  RotationMethod=StandardAxis  RotationAngleUnits=deg  RotationStandardAxis=+X  RotationAngle=1  RotationArbitraryAxis=[0 0 1]  FollAlignAxisA=+X  BaseAlignAxisA=+Y  FollAlignAxisB=+Y  BaseAlignAxisB=+Z  BlockFunction=simmechanics.library.frames_transforms.rigid_transform
  Rigid Transform7 : sm_lib/Frames and Transforms/Rigid Transform  TranslationMethod=Cartesian  TranslationLengthUnit=m  TranslationStandardAxis=+Z  TranslationStandardOffset=0  TranslationCartesianOffset=[5 -2 -0.55]  TranslationROffset=0  TranslationROffsetUnits=m  TranslationZOffset=0  TranslationZOffsetUnits=m  TranslationThetaOffset=0  TranslationThetaOffsetUnits=deg  RotationMethod=StandardAxis  RotationAngleUnits=deg  RotationStandardAxis=+Z  RotationAngle=0  RotationArbitraryAxis=[0 0 1]  FollAlignAxisA=+X  BaseAlignAxisA=+Y  FollAlignAxisB=+Y  BaseAlignAxisB=+Z  RotationMatrix=[1 0 0; 0 1 0; 0 0 1]  BlockFunction=simmechanics.library.frames_transforms.rigid_transform
  Rigid Transform8 : sm_lib/Frames and Transforms/Rigid Transform  TranslationMethod=None  TranslationLengthUnit=m  TranslationStandardAxis=+Z  TranslationStandardOffset=0  TranslationCartesianOffset=[0 0 -1.25]  TranslationROffset=0  TranslationROffsetUnits=m  TranslationZOffset=0  TranslationZOffsetUnits=m  TranslationThetaOffset=0  TranslationThetaOffsetUnits=deg  RotationMethod=StandardAxis  RotationAngleUnits=deg  RotationStandardAxis=+Y  RotationAngle=-4  RotationArbitraryAxis=[0 0 1]  FollAlignAxisA=+X  BaseAlignAxisA=+Y  FollAlignAxisB=+Y  BaseAlignAxisB=+Z  BlockFunction=simmechanics.library.frames_transforms.rigid_transform
  Rigid Transform9 : sm_lib/Frames and Transforms/Rigid Transform  TranslationMethod=None  TranslationLengthUnit=m  TranslationStandardAxis=+Z  TranslationStandardOffset=0  TranslationCartesianOffset=[0 0 -1.25]  TranslationROffset=0  TranslationROffsetUnits=m  TranslationZOffset=0  TranslationZOffsetUnits=m  TranslationThetaOffset=0  TranslationThetaOffsetUnits=deg  RotationMethod=StandardAxis  RotationAngleUnits=deg  RotationStandardAxis=+X  RotationAngle=5  RotationArbitraryAxis=[0 0 1]  FollAlignAxisA=+X  BaseAlignAxisA=+Y  FollAlignAxisB=+Y  BaseAlignAxisB=+Z  BlockFunction=simmechanics.library.frames_transforms.rigid_transform
  Solver Configuration : nesl_utility/Solver Configuration  PhysicalDomain=network_engine_domain  SubClassName=solver  LeftPortType=input  RightPortType=generic  Accelerate=off  Tones=[]  Harmonics=[]  SimulateNoise=off  Profile=off  UseLocalSampling=off  EnableSwitchedLinearOptims=on  FrequencyDomain=off  UseCCode=off  RelTol=0.001  AbsTol=1e-06  MinStep=1e-09  ToWorkspace=off  DoDC=off  ResidualTolerance=1e-09  UseLocalSolver=off  LocalSolverChoice=NE_BACKWARD_EULER_ADVANCER  LocalSolverSampleTime=0.001  DoFixedCost=off  MaxNonlinIter=3  MaxModeIter=2  LinearAlgebra=Sparse  DelaysMemoryBudget=1024  AutomaticFiltering=on  FilteringTimeConstant=0.001
  World Frame : sm_lib/Frames and Transforms/World Frame  BlockFunction=simmechanics.library.frames_transforms.world_frame
  LW : PMIOPort  Port=1  Side=Right
  wl : PMIOPort  Port=2  Side=Right
  RW : PMIOPort  Port=3  Side=Right
  wr : PMIOPort  Port=4  Side=Right
  Robot : PMIOPort  Port=5  Side=Left
  connections:
  Rigid Transform9/RConn1 -- Contact Force + Torque (2 Wheels)2/LConn1
  Rigid Transform8/LConn1 -- Rigid Transform7/RConn1
  Rigid Transform9/LConn1 -- Rigid Transform8/RConn1
  Contact Force + Torque (2 Wheels)/RConn1 -- Contact Force + Torque (2 Wheels)1/RConn1 -- Contact Force + Torque (2 Wheels)2/RConn1 -- LW/RConn1
  Rigid Transform5/LConn1 -- Rigid Transform4/RConn1
  Rigid Transform6/LConn1 -- Rigid Transform5/RConn1
  Rigid Transform6/RConn1 -- Contact Force + Torque (2 Wheels)1/LConn1
  Rigid Transform1/RConn1 -- Rigid Transform2/LConn1
  Rigid Transform3/RConn1 -- Rigid Transform1/LConn1
  Contact Force + Torque (2 Wheels)/RConn3 -- Contact Force + Torque (2 Wheels)1/RConn3 -- Contact Force + Torque (2 Wheels)2/RConn3 -- RW/RConn1
  Contact Force + Torque (2 Wheels)1/RConn2 -- Contact Force + Torque (2 Wheels)2/RConn2 -- Contact Force + Torque (2 Wheels)/RConn2 -- wl/RConn1
  Rigid Transform3/LConn1 -- Robot/RConn1 -- World Frame/RConn1 -- Rigid Transform4/LConn1 -- Mechanism Configuration/RConn1 -- Rigid Transform7/LConn1 -- Solver Configuration/RConn1
  Contact Force + Torque (2 Wheels)2/RConn4 -- Contact Force + Torque (2 Wheels)1/RConn4 -- Contact Force + Torque (2 Wheels)/RConn4 -- wr/RConn1
  Rigid Transform2/RConn1 -- Contact Force + Torque (2 Wheels)/LConn1
